simulink model "simulink_cpu_model"  (R2025b)
settings: Solver=FixedStepDiscrete  StartTime=0.0  StopTime=3  FixedStep=0.005  RelTol=1e-3
values from neighbouring files (symbols this model uses):
  u_input = zeros(num_channels, 1)    [compare_cpu_vs_gpu.m]    (also in diagnose_gpu_output.m = zeros(1024, 1))
settings Model: Creator=fbetancourt  LastModifiedBy=fbetancourt

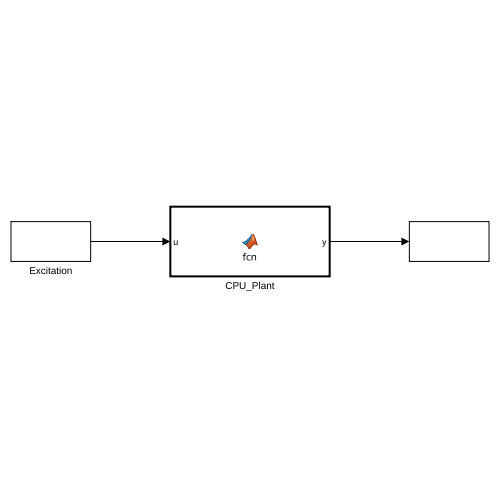
[thumbnail: Simulink's stored preview of the top-level diagram]
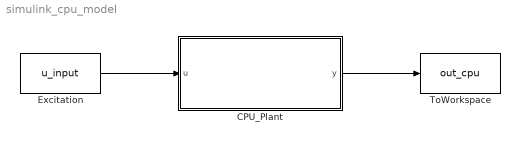
== system simulink_cpu_model ==
  CPU_Plant : MATLAB Function  TreatAsAtomicUnit=on
  Excitation : Constant  Value=u_input
  ToWorkspace : ToWorkspace  VariableName=out_cpu  SampleTime=-1
  wires:
  Excitation/1 -> CPU_Plant/1(u)
  CPU_Plant/1(y) -> ToWorkspace/1

== matlab function simulink_cpu_model/CPU_Plant ==
  data: u input; y output
function y = fcn(u)
persistent pos vel;
n = 1024;
dt = 0.005000;
damping = 0.050000;
k = 20.0;
if isempty(pos)
    pos = zeros(n, 1, 'single');
    vel = zeros(n, 1, 'single');
end
p_left  = [0; pos(1:end-1)];
p_right = [pos(2:end); 0];
force = single(u) - k * (2.0 * pos - p_left - p_right) - damping * vel;
vel = vel + force * dt;
pos = pos + vel * dt;
y = double(pos);
